simulink model "State_Machine_Harness_SignalBuilder"  (R2020b)
settings: Solver=FixedStepDiscrete  StartTime=0.0  StopTime=85  RelTol=1e-3  EnableMultiTasking=on
undefined symbols (not defined in the file): sigbuilder_block
settings Model: DataDictionary=DD_State_Machine.sldd  Creator=falderis  LastModifiedBy=lordx
settings SolverCC: AutoInsertRateTranBlk=on
settings DataIOCC: ExternalInput=Battery  SaveOutput=off  SaveTime=off  SignalLoggingName=logsOut
settings OptimizationCC: DefaultParameterBehavior=Inlined  UseDivisionForNetSlopeComputation=on  UseFloatMulNetSlope=on  DefaultUnderspecifiedDataType=single  UseSpecifiedMinMax=on  InlineInvariantSignals=on  PassReuseOutputArgsAs=Individual arguments  ZeroExternalMemoryAtStartup=off  ZeroInternalMemoryAtStartup=off  NoFixptDivByZeroProtection=on  EfficientFloat2IntCast=on  LifeSpan=inf  MaxStackSize=64  OptimizeBlockOrder=speed  DifferentSizesBufferReuse=on  EfficientTunableParamExpr=on
settings DebuggingCC: SignalInfNanChecking=error  SaveWithParameterizedLinksMsg=none  UnderspecifiedInitializationDetection=Classic  MergeDetectMultiDrivingBlocksExec=none  CheckExecutionContextPreStartOutputMsg=on  CheckExecutionContextRuntimeOutputMsg=on  IntegerOverflowMsg=error  ParameterPrecisionLossMsg=none  ParameterTunabilityLossMsg=error  AssertControl=DisableAll  PregeneratedLibrarySubsystemCodeDiagnostic=none  SFUnexpectedBacktrackingDiag=warning  SFNoUnconditionalDefaultTransitionDiag=warning  SFExecutionAtInitializationDiag=none  ArithmeticOperatorsInVariantConditions=warning
settings HardwareCC: ProdBitPerPointer=32  ProdBitPerSizeT=32  ProdBitPerPtrDiffT=32  ProdLargestAtomicFloat=None  ProdWordSize=32  ProdHWDeviceType=Custom Processor->Custom Processor
settings ModelReferenceCC: ModelReferenceNumInstancesAllowed=Single  PropagateSignalLabelsOutOfModel=off
settings SFSimCC: SimUseLocalCustomCode=off  MATLABDynamicMemAlloc=off  CustomCodeUndefinedFunction=UseInterfaceOnly
settings RTWCC: Description=Embedded Coder  SystemTargetFile=ert.tlc  GenCodeOnly=on  TemplateMakefile=ert_default_tmf  GenerateReport=on  RTWUseLocalCustomCode=off  IncludeHyperlinkInReport=on  GenerateTraceInfo=on  GenerateTraceReport=on  GenerateTraceReportSl=on  GenerateTraceReportSf=on  GenerateTraceReportEml=on  GenerateWebview=on  GenerateCodeMetricsReport=on
settings CodeAppCC: ForceParamTrailComments=on  IgnoreCustomStorageClasses=off  MaxIdLength=51  OperatorAnnotations=on  SimulinkDataObjDesc=on  SFDataObjDesc=on  MangleLength=4  InsertBlockDesc=on  ReqsInCode=on
settings ERTTargetCC: UtilityFuncGeneration=Shared location  GenerateSampleERTMain=on  IncludeMdlTerminateFcn=off  CombineSignalStateStructs=on  SuppressErrorStatus=on  SupportNonFinite=off  SupportComplex=off  ParenthesesLevel=Maximum  CastingMode=Standards  GenerateSharedConstants=off  InlinedParameterPlacement=NonHierarchical  ERTCustomFileTemplate=example_file_process.tlc  PreserveExpressionOrder=on  PreserveIfCondition=on  EnableSignedLeftShifts=off  EnableSignedRightShifts=off
settings ConfigComp: CovScope=ReferencedModels  CovIncludeTopModel=off  CovMetricSettings=dcw  CovSaveCumulativeToWorkspaceVar=on  CovSaveSingleToWorkspaceVar=on  CovExternalEMLEnable=off  CovSFcnEnable=off  DVMode=DesignErrorDetection  DVMaxProcessTime=7000  DVTestSuiteOptimization=Auto  DVDetectDeadLogic=on  DVDetectIntegerOverflow=off  DVRebuildModelRepresentation=Always

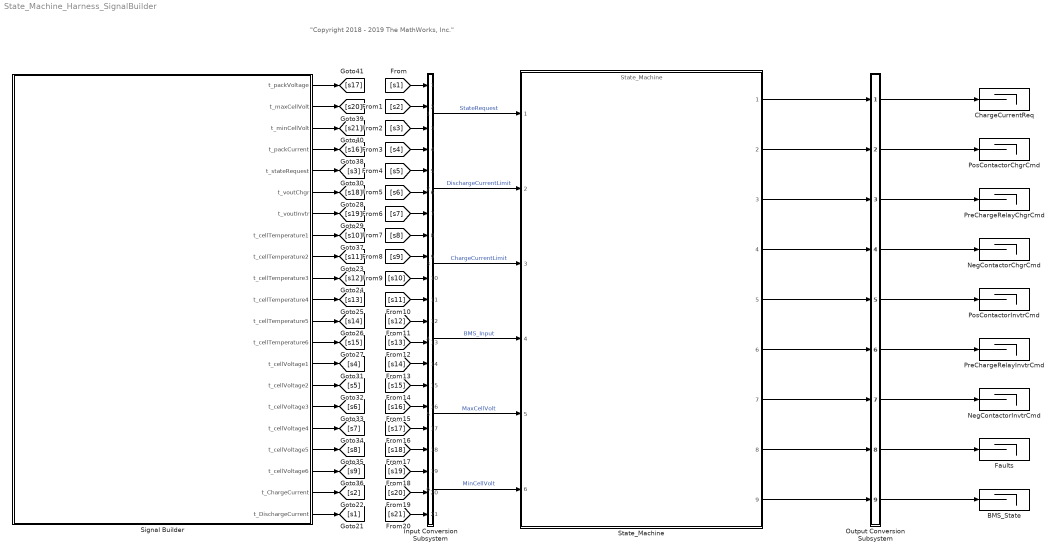
== system State_Machine_Harness_SignalBuilder ==
  note: "Copyright 2018 - 2019 The MathWorks, Inc."
  BMS_State : Terminator
  ChargeCurrentReq : Terminator
  Faults : Terminator
  Input Conversion Subsystem : Subsystem  Tag=__SLT_ICS__  Description=|
      | Signal spec.
      | and routing
      settings: AttributesFormatString=%<Description>
  NegContactorChgrCmd : Terminator
  NegContactorInvtrCmd : Terminator
  Output Conversion Subsystem : Subsystem  Tag=__SLT_OCS__  Description=|
      | Signal spec.
      | and routing
      settings: AttributesFormatString=%<Description>
  PosContactorChgrCmd : Terminator
  PosContactorInvtrCmd : Terminator
  PreChargeRelayChgrCmd : Terminator
  PreChargeRelayInvtrCmd : Terminator
  Signal Builder : Subsystem  Tag=STV Subsys  LoadFcn=sigbuilder_block('load');  StartFcn=sigbuilder_block('start');  StopFcn=sigbuilder_block('stop');  ClipboardFcn=sigbuilder_block('clipboard');  mask(Sigbuilder block){tuvar=[0:10]}
      mask help: Simulink:masks:SigbuilderBlock_MD
      mask init:
      | if ~strcmp(get_param(bdroot(gcbh),'SimulationStatus'),'stopped') tuvar = sigbuilder_block('maskInit'); end
      settings: CopyFcn=sigbuilder_block('copy');  DeleteFcn=sigbuilder_block('delete');  ModelCloseFcn=sigbuilder_block('modelClose');  PreSaveFcn=sigbuilder_block('preSave');  PauseFcn=sigbuilder_block('pause');  ContinueFcn=sigbuilder_block('continue');  NameChangeFcn=sigbuilder_block('namechange');  OpenFcn=sigbuilder_block('open',[1962.75 -162.75 1043.25 773.25 ]);  CloseFcn=sigbuilder_block('close');
      mask Display: plot(0, 0, 100, 100,[2, 2, 32, 32, 2], [68, 8, 8, 68, 68],[32, 2], [38, 38], [32, 19, 2],[53, 60, 44], [32, 17, 17, 2],[16, 16, 31, 31]);txt = getActiveGroup(gcbh);text(2, 100, txt,'verticalAlignment', 'top');
  State_Machine : ModelReference  ModelNameDialog=State_Machine  SimulationMode=Normal  ModelReferenceVersion=1.671
  wires:
  Output Conversion Subsystem/1(Outport_1) -> ChargeCurrentReq/1
  Output Conversion Subsystem/2(Outport_2) -> PosContactorChgrCmd/1
  Output Conversion Subsystem/3(Outport_3) -> PreChargeRelayChgrCmd/1
  Output Conversion Subsystem/4(Outport_4) -> NegContactorChgrCmd/1
  Output Conversion Subsystem/5(Outport_5) -> PosContactorInvtrCmd/1
  Output Conversion Subsystem/6(Outport_6) -> PreChargeRelayInvtrCmd/1
  Output Conversion Subsystem/7(Outport_7) -> NegContactorInvtrCmd/1
  Output Conversion Subsystem/8(Outport_8) -> Faults/1
  Output Conversion Subsystem/9(Outport_9) -> BMS_State/1
  State_Machine/1 -> Output Conversion Subsystem/1(Inport_1)
  State_Machine/2 -> Output Conversion Subsystem/2(Inport_2)
  State_Machine/3 -> Output Conversion Subsystem/3(Inport_3)
  State_Machine/4 -> Output Conversion Subsystem/4(Inport_4)
  State_Machine/5 -> Output Conversion Subsystem/5(Inport_5)
  State_Machine/6 -> Output Conversion Subsystem/6(Inport_6)
  State_Machine/7 -> Output Conversion Subsystem/7(Inport_7)
  State_Machine/8 -> Output Conversion Subsystem/8(Inport_8)
  State_Machine/9 -> Output Conversion Subsystem/9(Inport_9)
  [s1] -> Input Conversion Subsystem/1(Inport_1)
  [s2] -> Input Conversion Subsystem/2(Inport_2)
  [s3] -> Input Conversion Subsystem/3(Inport_3)
  [s4] -> Input Conversion Subsystem/4(Inport_4)
  [s5] -> Input Conversion Subsystem/5(Inport_5)
  [s6] -> Input Conversion Subsystem/6(Inport_6)
  [s7] -> Input Conversion Subsystem/7(Inport_7)
  [s8] -> Input Conversion Subsystem/8(Inport_8)
  [s9] -> Input Conversion Subsystem/9(Inport_9)
  [s10] -> Input Conversion Subsystem/10(Inport_10)
  [s11] -> Input Conversion Subsystem/11(Inport_11)
  [s12] -> Input Conversion Subsystem/12(Inport_12)
  [s13] -> Input Conversion Subsystem/13(Inport_13)
  [s14] -> Input Conversion Subsystem/14(Inport_14)
  [s15] -> Input Conversion Subsystem/15(Inport_15)
  [s16] -> Input Conversion Subsystem/16(Inport_16)
  [s17] -> Input Conversion Subsystem/17(Inport_17)
  [s18] -> Input Conversion Subsystem/18(Inport_18)
  [s19] -> Input Conversion Subsystem/19(Inport_19)
  [s20] -> Input Conversion Subsystem/20(Inport_20)
  [s21] -> Input Conversion Subsystem/21(Inport_21)
  Signal Builder/5(t_stateRequest) -> [s3]
  Signal Builder/1(t_packVoltage) -> [s17]
  Signal Builder/2(t_maxCellVolt) -> [s20]
  Signal Builder/3(t_minCellVolt) -> [s21]
  Signal Builder/4(t_packCurrent) -> [s16]
  Signal Builder/6(t_voutChgr) -> [s18]
  Signal Builder/7(t_voutInvtr) -> [s19]
  Signal Builder/8(t_cellTemperature1) -> [s10]
  Signal Builder/9(t_cellTemperature2) -> [s11]
  Signal Builder/10(t_cellTemperature3) -> [s12]
  Signal Builder/11(t_cellTemperature4) -> [s13]
  Signal Builder/12(t_cellTemperature5) -> [s14]
  Signal Builder/13(t_cellTemperature6) -> [s15]
  Signal Builder/14(t_cellVoltage1) -> [s4]
  Signal Builder/15(t_cellVoltage2) -> [s5]
  Signal Builder/16(t_cellVoltage3) -> [s6]
  Signal Builder/17(t_cellVoltage4) -> [s7]
  Signal Builder/18(t_cellVoltage5) -> [s8]
  Signal Builder/19(t_cellVoltage6) -> [s9]
  Signal Builder/20(t_ChargeCurrent) -> [s2]
  Signal Builder/21(t_DischargeCurrent) -> [s1]
  Input Conversion Subsystem/6(Outport_10) -> State_Machine/6  "MinCellVolt"
  Input Conversion Subsystem/5(Outport_9) -> State_Machine/5  "MaxCellVolt"
  Input Conversion Subsystem/1(Outport_2) -> State_Machine/1  "StateRequest"
  Input Conversion Subsystem/2(Outport_1) -> State_Machine/2  "DischargeCurrentLimit"
  Input Conversion Subsystem/3(Outport_11) -> State_Machine/3  "ChargeCurrentLimit"
  Input Conversion Subsystem/4(Outport_3) -> State_Machine/4  "BMS_Input"

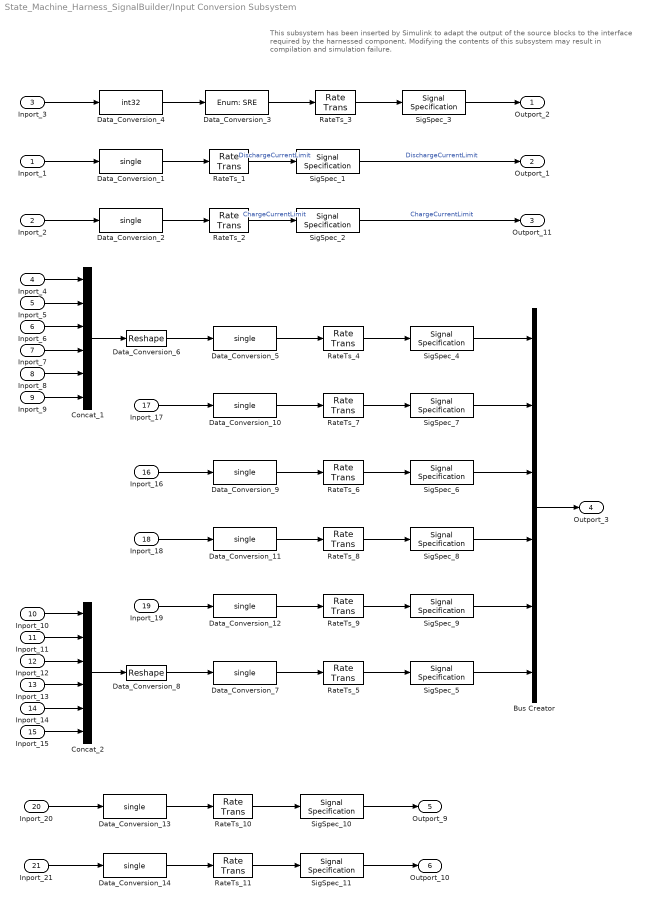
== system State_Machine_Harness_SignalBuilder/Input Conversion Subsystem ==
  note: This subsystem has been inserted by Simulink to adapt the output of the source blocks to the interface required by the harnessed component.
      |  Modifying the contents of this subsystem may result in compilation and simulation failure.
  Inport_1 : Inport
  Inport_2 : Inport  Port=2
  Inport_3 : Inport  Port=3
  Inport_4 : Inport  Port=4
  Inport_5 : Inport  Port=5
  Inport_6 : Inport  Port=6
  Inport_7 : Inport  Port=7
  Inport_8 : Inport  Port=8
  Inport_9 : Inport  Port=9
  Inport_10 : Inport  Port=10
  Inport_11 : Inport  Port=11
  Inport_12 : Inport  Port=12
  Inport_13 : Inport  Port=13
  Inport_14 : Inport  Port=14
  Inport_15 : Inport  Port=15
  Inport_16 : Inport  Port=16
  Inport_17 : Inport  Port=17
  Inport_18 : Inport  Port=18
  Inport_19 : Inport  Port=19
  Inport_20 : Inport  Port=20
  Inport_21 : Inport  Port=21
  Bus Creator : BusCreator  Inputs=6  OutDataTypeStr=Bus: BMS_Input
      settings: InheritFromInputs=off
  Concat_1 : Concatenate  NumInputs=6
  Concat_2 : Concatenate  NumInputs=6
  Data_Conversion_{1..2,5,7,9..14} (10 alike) : DataTypeConversion  OutDataTypeStr=single  SaturateOnIntegerOverflow=on  RndMeth=Zero
  Data_Conversion_3 : DataTypeConversion  OutDataTypeStr=Enum: SRE  SaturateOnIntegerOverflow=on  RndMeth=Zero
  Data_Conversion_4 : DataTypeConversion  OutDataTypeStr=int32  RndMeth=Round  SaturateOnIntegerOverflow=on
  Data_Conversion_6 : Reshape  OutputDimensionality=Customize  OutputDimensions=[6]
  Data_Conversion_8 : Reshape  OutputDimensionality=Customize  OutputDimensions=[6]
  RateTs_{1..11} (11 alike) : RateTransition  OutPortSampleTime=0.1
  SigSpec_{1..2,6..11} (8 alike) : SignalSpecification  OutDataTypeStr=single  Dimensions=[1]  SampleTime=0.1
  SigSpec_3 : SignalSpecification  OutDataTypeStr=Enum: SRE  Dimensions=[1]  SampleTime=0.1
  SigSpec_4 : SignalSpecification  OutDataTypeStr=single  Dimensions=[6]  SampleTime=0.1
  SigSpec_5 : SignalSpecification  OutDataTypeStr=single  Dimensions=[6]  SampleTime=0.1
  Outport_2 : Outport  VectorParamsAs1DForOutWhenUnconnected=off
  Outport_1 : Outport  Port=2  VectorParamsAs1DForOutWhenUnconnected=off
  Outport_11 : Outport  Port=3  VectorParamsAs1DForOutWhenUnconnected=off
  Outport_3 : Outport  Port=4  VectorParamsAs1DForOutWhenUnconnected=off
  Outport_9 : Outport  Port=5  VectorParamsAs1DForOutWhenUnconnected=off
  Outport_10 : Outport  Port=6  VectorParamsAs1DForOutWhenUnconnected=off
  wires:
  SigSpec_1/1 -> Outport_1/1  "DischargeCurrentLimit"
  RateTs_1/1 -> SigSpec_1/1  "DischargeCurrentLimit"
  Data_Conversion_1/1 -> RateTs_1/1
  Inport_1/1 -> Data_Conversion_1/1
  SigSpec_2/1 -> Outport_11/1  "ChargeCurrentLimit"
  RateTs_2/1 -> SigSpec_2/1  "ChargeCurrentLimit"
  Data_Conversion_2/1 -> RateTs_2/1
  Inport_2/1 -> Data_Conversion_2/1
  SigSpec_3/1 -> Outport_2/1
  RateTs_3/1 -> SigSpec_3/1
  Data_Conversion_3/1 -> RateTs_3/1
  Data_Conversion_4/1 -> Data_Conversion_3/1
  Inport_3/1 -> Data_Conversion_4/1
  RateTs_4/1 -> SigSpec_4/1
  Data_Conversion_5/1 -> RateTs_4/1
  Data_Conversion_6/1 -> Data_Conversion_5/1
  Concat_1/1 -> Data_Conversion_6/1
  Inport_4/1 -> Concat_1/1
  Inport_5/1 -> Concat_1/2
  Inport_6/1 -> Concat_1/3
  Inport_7/1 -> Concat_1/4
  Inport_8/1 -> Concat_1/5
  Inport_9/1 -> Concat_1/6
  SigSpec_5/1 -> Bus Creator/6
  RateTs_5/1 -> SigSpec_5/1
  Data_Conversion_7/1 -> RateTs_5/1
  Data_Conversion_8/1 -> Data_Conversion_7/1
  Concat_2/1 -> Data_Conversion_8/1
  Inport_10/1 -> Concat_2/1
  Inport_11/1 -> Concat_2/2
  Inport_12/1 -> Concat_2/3
  Inport_13/1 -> Concat_2/4
  Inport_14/1 -> Concat_2/5
  Inport_15/1 -> Concat_2/6
  SigSpec_6/1 -> Bus Creator/3
  RateTs_6/1 -> SigSpec_6/1
  Data_Conversion_9/1 -> RateTs_6/1
  Inport_16/1 -> Data_Conversion_9/1
  SigSpec_7/1 -> Bus Creator/2
  RateTs_7/1 -> SigSpec_7/1
  Data_Conversion_10/1 -> RateTs_7/1
  Inport_17/1 -> Data_Conversion_10/1
  SigSpec_8/1 -> Bus Creator/4
  RateTs_8/1 -> SigSpec_8/1
  Data_Conversion_11/1 -> RateTs_8/1
  Inport_18/1 -> Data_Conversion_11/1
  SigSpec_9/1 -> Bus Creator/5
  RateTs_9/1 -> SigSpec_9/1
  Data_Conversion_12/1 -> RateTs_9/1
  Inport_19/1 -> Data_Conversion_12/1
  SigSpec_10/1 -> Outport_9/1
  RateTs_10/1 -> SigSpec_10/1
  Data_Conversion_13/1 -> RateTs_10/1
  Inport_20/1 -> Data_Conversion_13/1
  SigSpec_11/1 -> Outport_10/1
  RateTs_11/1 -> SigSpec_11/1
  Data_Conversion_14/1 -> RateTs_11/1
  Inport_21/1 -> Data_Conversion_14/1
  SigSpec_4/1 -> Bus Creator/1
  Bus Creator/1 -> Outport_3/1

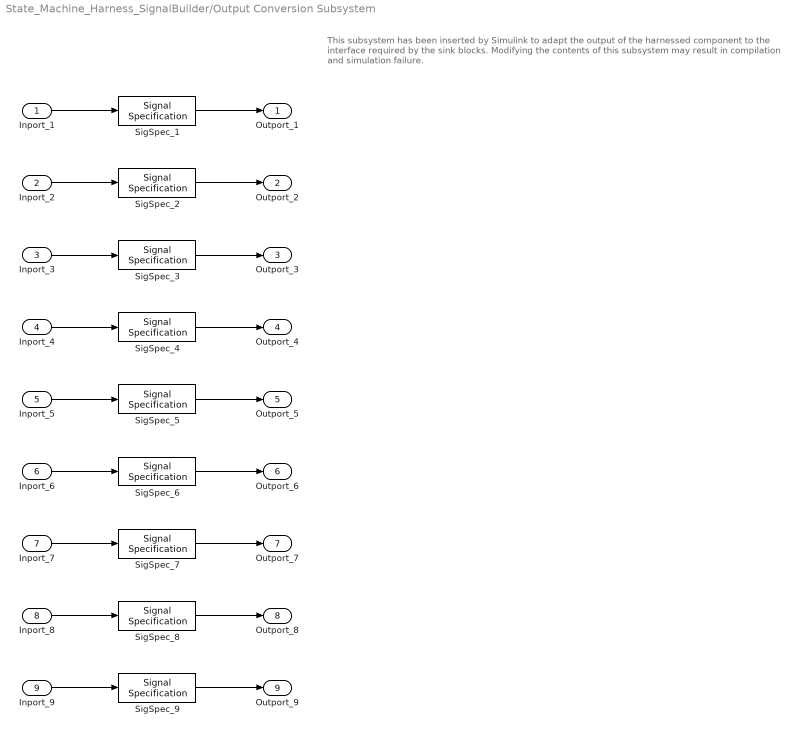
== system State_Machine_Harness_SignalBuilder/Output Conversion Subsystem ==
  note: This subsystem has been inserted by Simulink to adapt the output of the harnessed component to the interface required by the sink blocks.
      |  Modifying the contents of this subsystem may result in compilation and simulation failure.
  Inport_1 : Inport
  Inport_2 : Inport  Port=2
  Inport_3 : Inport  Port=3
  Inport_4 : Inport  Port=4
  Inport_5 : Inport  Port=5
  Inport_6 : Inport  Port=6
  Inport_7 : Inport  Port=7
  Inport_8 : Inport  Port=8
  Inport_9 : Inport  Port=9
  SigSpec_1 : SignalSpecification  OutDataTypeStr=single  Dimensions=[1]  SampleTime=0.1
  SigSpec_{2..7} (6 alike) : SignalSpecification  OutDataTypeStr=boolean  Dimensions=[1]  SampleTime=0.1
  SigSpec_8 : SignalSpecification  OutDataTypeStr=Bus: Faults  Dimensions=[1]  SampleTime=0.1  BusOutputAsStruct=on
  SigSpec_9 : SignalSpecification  OutDataTypeStr=Enum: BMS_State_Enum  Dimensions=[1]  SampleTime=0.1
  Outport_1 : Outport  VectorParamsAs1DForOutWhenUnconnected=off
  Outport_2 : Outport  Port=2  VectorParamsAs1DForOutWhenUnconnected=off
  Outport_3 : Outport  Port=3  VectorParamsAs1DForOutWhenUnconnected=off
  Outport_4 : Outport  Port=4  VectorParamsAs1DForOutWhenUnconnected=off
  Outport_5 : Outport  Port=5  VectorParamsAs1DForOutWhenUnconnected=off
  Outport_6 : Outport  Port=6  VectorParamsAs1DForOutWhenUnconnected=off
  Outport_7 : Outport  Port=7  VectorParamsAs1DForOutWhenUnconnected=off
  Outport_8 : Outport  Port=8  VectorParamsAs1DForOutWhenUnconnected=off
  Outport_9 : Outport  Port=9  VectorParamsAs1DForOutWhenUnconnected=off
  wires:
  Inport_1/1 -> SigSpec_1/1
  SigSpec_1/1 -> Outport_1/1
  Inport_2/1 -> SigSpec_2/1
  SigSpec_2/1 -> Outport_2/1
  Inport_3/1 -> SigSpec_3/1
  SigSpec_3/1 -> Outport_3/1
  Inport_4/1 -> SigSpec_4/1
  SigSpec_4/1 -> Outport_4/1
  Inport_5/1 -> SigSpec_5/1
  SigSpec_5/1 -> Outport_5/1
  Inport_6/1 -> SigSpec_6/1
  SigSpec_6/1 -> Outport_6/1
  Inport_7/1 -> SigSpec_7/1
  SigSpec_7/1 -> Outport_7/1
  Inport_8/1 -> SigSpec_8/1
  SigSpec_8/1 -> Outport_8/1
  Inport_9/1 -> SigSpec_9/1
  SigSpec_9/1 -> Outport_9/1

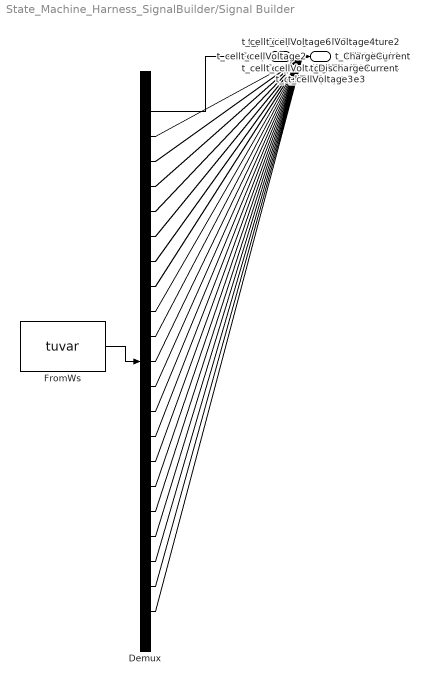
== system State_Machine_Harness_SignalBuilder/Signal Builder ==
  Demux : Demux  Tag=STV Demux  Outputs=21
      settings: DisplayOption=none
  FromWs : FromWorkspace  Tag=STV FromWs  VariableName=tuvar
  t_packVoltage : Outport  Tag=STV Outport  VectorParamsAs1DForOutWhenUnconnected=off
  t_maxCellVolt : Outport  Tag=STV Outport  Port=2  VectorParamsAs1DForOutWhenUnconnected=off
  t_minCellVolt : Outport  Tag=STV Outport  Port=3  VectorParamsAs1DForOutWhenUnconnected=off
  t_packCurrent : Outport  Tag=STV Outport  Port=4  VectorParamsAs1DForOutWhenUnconnected=off
  t_stateRequest : Outport  Tag=STV Outport  Port=5  VectorParamsAs1DForOutWhenUnconnected=off
  t_voutChgr : Outport  Tag=STV Outport  Port=6  VectorParamsAs1DForOutWhenUnconnected=off
  t_voutInvtr : Outport  Tag=STV Outport  Port=7  VectorParamsAs1DForOutWhenUnconnected=off
  t_cellTemperature1 : Outport  Tag=STV Outport  Port=8  VectorParamsAs1DForOutWhenUnconnected=off
  t_cellTemperature2 : Outport  Tag=STV Outport  Port=9  VectorParamsAs1DForOutWhenUnconnected=off
  t_cellTemperature3 : Outport  Tag=STV Outport  Port=10  VectorParamsAs1DForOutWhenUnconnected=off
  t_cellTemperature4 : Outport  Tag=STV Outport  Port=11  VectorParamsAs1DForOutWhenUnconnected=off
  t_cellTemperature5 : Outport  Tag=STV Outport  Port=12  VectorParamsAs1DForOutWhenUnconnected=off
  t_cellTemperature6 : Outport  Tag=STV Outport  Port=13  VectorParamsAs1DForOutWhenUnconnected=off
  t_cellVoltage1 : Outport  Tag=STV Outport  Port=14  VectorParamsAs1DForOutWhenUnconnected=off
  t_cellVoltage2 : Outport  Tag=STV Outport  Port=15  VectorParamsAs1DForOutWhenUnconnected=off
  t_cellVoltage3 : Outport  Tag=STV Outport  Port=16  VectorParamsAs1DForOutWhenUnconnected=off
  t_cellVoltage4 : Outport  Tag=STV Outport  Port=17  VectorParamsAs1DForOutWhenUnconnected=off
  t_cellVoltage5 : Outport  Tag=STV Outport  Port=18  VectorParamsAs1DForOutWhenUnconnected=off
  t_cellVoltage6 : Outport  Tag=STV Outport  Port=19  VectorParamsAs1DForOutWhenUnconnected=off
  t_ChargeCurrent : Outport  Tag=STV Outport  Port=20  VectorParamsAs1DForOutWhenUnconnected=off
  t_DischargeCurrent : Outport  Tag=STV Outport  Port=21  VectorParamsAs1DForOutWhenUnconnected=off
  wires:
  Demux/1 -> t_packVoltage/1
  FromWs/1 -> Demux/1
  Demux/2 -> t_maxCellVolt/1
  Demux/3 -> t_minCellVolt/1
  Demux/4 -> t_packCurrent/1
  Demux/5 -> t_stateRequest/1
  Demux/6 -> t_voutChgr/1
  Demux/7 -> t_voutInvtr/1
  Demux/8 -> t_cellTemperature1/1
  Demux/9 -> t_cellTemperature2/1
  Demux/10 -> t_cellTemperature3/1
  Demux/11 -> t_cellTemperature4/1
  Demux/12 -> t_cellTemperature5/1
  Demux/13 -> t_cellTemperature6/1
  Demux/14 -> t_cellVoltage1/1
  Demux/15 -> t_cellVoltage2/1
  Demux/16 -> t_cellVoltage3/1
  Demux/17 -> t_cellVoltage4/1
  Demux/18 -> t_cellVoltage5/1
  Demux/19 -> t_cellVoltage6/1
  Demux/20 -> t_ChargeCurrent/1
  Demux/21 -> t_DischargeCurrent/1
